simulink model "ex_pend_free"  (R2023a)
settings: Solver=ode2  StartTime=0.0  StopTime=30  FixedStep=h  RelTol=1e-3  EnableMultiTasking=on
libraries: carterlib x1
settings Model: ExtModeTrigDuration=2  Creator=kawata  LastModifiedBy=kawata
settings SolverCC: AutoInsertRateTranBlk=on
settings DataIOCC: ReturnWorkspaceOutputs=off
settings OptimizationCC: DefaultParameterBehavior=Inlined  EnhancedBackFolding=on  PassReuseOutputArgsAs=Individual arguments  ZeroExternalMemoryAtStartup=off  ZeroInternalMemoryAtStartup=off  MaxStackSize=64  OptimizeBlockOrder=speed  DifferentSizesBufferReuse=on  OptimizationCustomize=off  EfficientTunableParamExpr=on
settings DebuggingCC: ParameterTunabilityLossMsg=error
settings HardwareCC: ProdBitPerInt=16  ProdBitPerPointer=16  ProdBitPerSizeT=16  ProdBitPerPtrDiffT=16  ProdLargestAtomicFloat=None  ProdWordSize=8  ProdHWDeviceType=Atmel->AVR  UseEmbeddedCoderFeatures=off
settings SFSimCC: MATLABDynamicMemAlloc=off
settings RTWCC: Description=Embedded Coder  SystemTargetFile=ert.tlc  HardwareBoard=Arduino Mega 2560  TemplateMakefile=ert_default_tmf  Toolchain=Arduino AVR  BuildConfiguration=Faster Runs  GPUComputeCapability=5.0
settings CodeAppCC: ForceParamTrailComments=on  IgnoreCustomStorageClasses=off  OperatorAnnotations=on  SimulinkDataObjDesc=on  SFDataObjDesc=on  InsertBlockDesc=on
settings ERTTargetCC: SupportContinuousTime=on  SupportNonInlinedSFcns=on  SupportVariableSizeSignals=on  ExtModeTransport=3  ExtModeStaticAlloc=on  ExtModeAutomaticAllocSize=off  ExtModeStaticAllocSize=2048  ExtModeMexFile=ext_xcp  ExtModeIntrfLevel=Level2 - Open  InlinedParameterPlacement=NonHierarchical

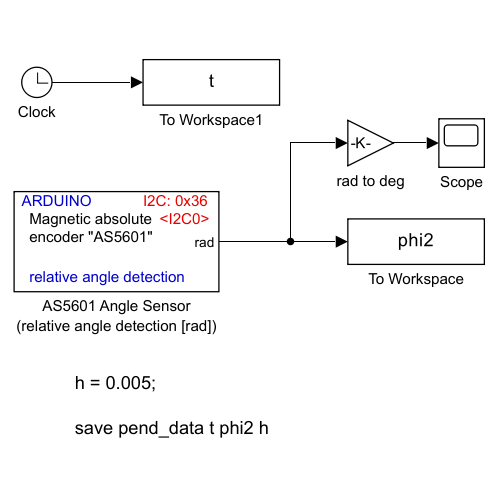
[thumbnail: Simulink's stored preview of the top-level diagram]
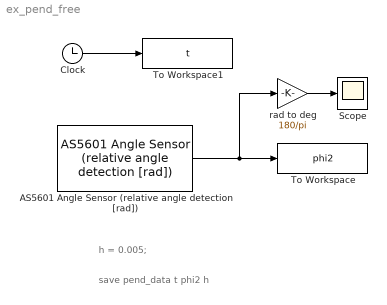
== system ex_pend_free ==
  note: h = 0.005;
  note: save pend_data t phi2 h
  AS5601 Angle Sensor (relative angle detection [rad]) : carterlib/AS5601 Angle Sensor (relative angle detection [rad])  sample_time=-1  I2CModule=0
  Clock : Clock
  Scope : Scope
  To Workspace : ToWorkspace  VariableName=phi2  SampleTime=-1
  To Workspace1 : ToWorkspace  VariableName=t  SampleTime=-1
  rad to deg : Gain  Gain=180/pi
  wires:
  AS5601 Angle Sensor (relative angle detection [rad])/1 -> rad to deg/1, To Workspace/1
  Clock/1 -> To Workspace1/1
  rad to deg/1 -> Scope/1
